simulink model "VIPL557StEnCtrl"  (R2018b)
settings: Solver=FixedStepDiscrete  StartTime=0.0  StopTime=10.0  FixedStep=0.01  RelTol=1e-3
undefined symbols (not defined in the file): data, KeSMSw4SSecRwLtStLgrstUpwdDnwdOpenPos1_Val, SecRwLtStBkReclnEn_Clear, SecRwLtStBkReclnEn_Set, SecRwLtStFwdBkwdEn_Clear, SecRwLtStFwdBkwdEn_Set, SecRwLtStLgrstInwdOtwdEn_Clear, SecRwLtStLgrstInwdOtwdEn_Set, SecRwLtStLgrstUpwdDnwdEn_Clear, SecRwLtStLgrstUpwdDnwdEn_Set, ThdRwLtStBkReclnEn_Clear, ThdRwLtStBkReclnEn_Set, ThdRwLtStFwdBkwdEn_Clear, ThdRwLtStFwdBkwdEn_Set, ZeroLEn_Clear, ZeroLEn_Set
libraries: simulink x1
settings Model: Creator=sn2xws  LastModifiedBy=sn2xws
settings Model: ModifiedHistory=|
  | 2024.7.2 V3.0.0 557模式流程V1.9
  | 2024.8.16 V3.0.1目标位置改为立即获取
  | 2024.8.22 V3.0.2 增加FirstTrig参数，智享目标位置计算改为只调用一次
  | 2024.8.30 V3.0.3 修复第一次会退出的问题
  | 2025.6.25 V3.13.0 Bug 1068643 偶发腿托及延伸先打开后动前后的问题
settings DataIOCC: SaveFormat=StructureWithTime
settings OptimizationCC: DefaultParameterBehavior=Inlined  EnhancedBackFolding=on  PassReuseOutputArgsAs=Individual arguments  ZeroExternalMemoryAtStartup=off  ZeroInternalMemoryAtStartup=off  OptimizeBlockOrder=speed  DifferentSizesBufferReuse=on  OptimizationCustomize=off
settings DebuggingCC: ParameterTunabilityLossMsg=error
settings SFSimCC: MATLABDynamicMemAlloc=off
settings RTWCC: SystemTargetFile=autosar.tlc  GenCodeOnly=on  TemplateMakefile=ert_default_tmf  Description=AUTOSAR  GenerateReport=on  IncludeHyperlinkInReport=on  LaunchReport=on  GenerateTraceInfo=on  GenerateTraceReport=on  GenerateTraceReportSl=on  GenerateTraceReportSf=on  GenerateTraceReportEml=on
settings CodeAppCC: ForceParamTrailComments=on  IgnoreCustomStorageClasses=off  OperatorAnnotations=on  SimulinkDataObjDesc=on  SFDataObjDesc=on  InsertBlockDesc=on
settings STFCustomTargetCC: TargetLangStandard=C99 (ISO)  MultiwordLength=256  ParMdlRefBuildCompliant=on  CompOptLevelCompliant=on  IncludeMdlTerminateFcn=off  CombineOutputUpdateFcns=on  SuppressErrorStatus=on  ERTCustomFileBanners=on  SupportNonFinite=off  SupportComplex=off  SupportContinuousTime=off  SupportNonInlinedSFcns=off  RemoveResetFunc=on  MATLABClassNameForMDSCustomization=Simulink.SoftwareTarget.ERTCustomization  AutosarCompliant=on  UseToolchainInfoCompliant=on  LookupTableObjectStructAxisOrder=2,1,3,4,...  LUTObjectStructOrderEvenSpacing=Size,Table,Breakpoints  SystemTargetFile=autosar.tlc
settings ERTTargetCC: TargetLangStandard=C99 (ISO)  ConcurrentExecutionCompliant=off  IncludeMdlTerminateFcn=off  SuppressErrorStatus=on  SupportNonFinite=off  SupportComplex=off  ModelStepFunctionPrototypeControlCompliant=off  CPPClassGenCompliant=off  AutosarCompliant=on  LookupTableObjectStructAxisOrder=2,1,3,4,...  LUTObjectStructOrderEvenSpacing=Size,Table,Breakpoints  InlinedParameterPlacement=NonHierarchical  ERTCustomFileTemplate=example_file_process.tlc  ERTFilePackagingFormat=Compact

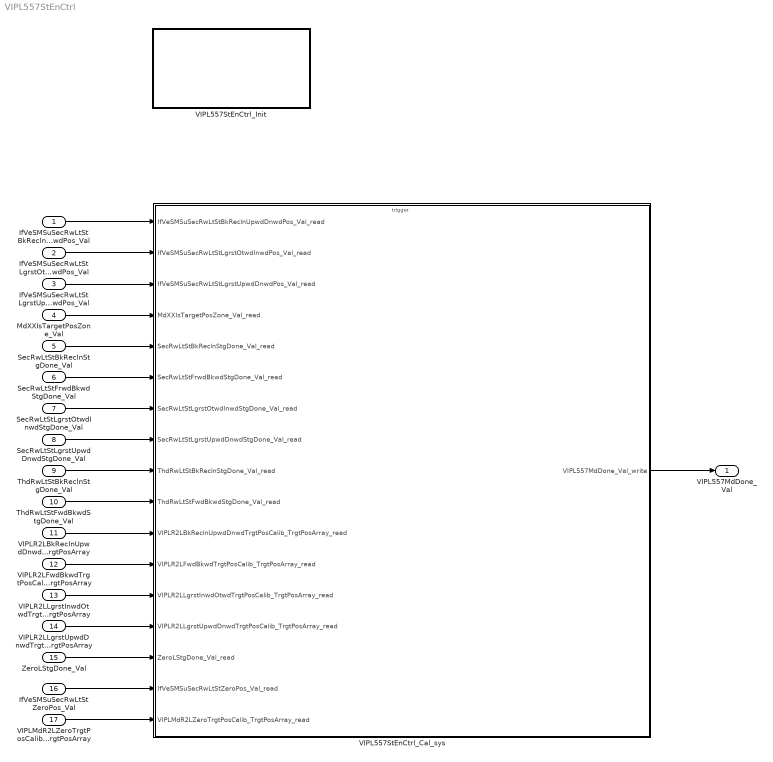
== system VIPL557StEnCtrl ==
  IfVeSMSuSecRwLtStBkReclnUpwdDnwdPos_Val : Inport  OutDataTypeStr=uint16  PortDimensions=1
  IfVeSMSuSecRwLtStLgrstOtwdInwdPos_Val : Inport  Port=2  OutDataTypeStr=uint16  PortDimensions=1
  IfVeSMSuSecRwLtStLgrstUpwdDnwdPos_Val : Inport  Port=3  OutDataTypeStr=uint16  PortDimensions=1
  MdXXIsTargetPosZone_Val : Inport  Port=4  OutDataTypeStr=uint32  PortDimensions=1
  SecRwLtStBkReclnStgDone_Val : Inport  Port=5  OutDataTypeStr=boolean  PortDimensions=1
  SecRwLtStFrwdBkwdStgDone_Val : Inport  Port=6  OutDataTypeStr=boolean  PortDimensions=1
  SecRwLtStLgrstOtwdInwdStgDone_Val : Inport  Port=7  OutDataTypeStr=boolean  PortDimensions=1
  SecRwLtStLgrstUpwdDnwdStgDone_Val : Inport  Port=8  OutDataTypeStr=boolean  PortDimensions=1
  ThdRwLtStBkReclnStgDone_Val : Inport  Port=9  OutDataTypeStr=boolean  PortDimensions=1
  ThdRwLtStFwdBkwdStgDone_Val : Inport  Port=10  OutDataTypeStr=boolean  PortDimensions=1
  VIPLR2LBkReclnUpwdDnwdTrgtPosCalib_TrgtPosArray : Inport  Description=|  Port=11  OutDataTypeStr=uint16  PortDimensions=3
      | 0:Pos
      | 1:Max
      | 2:Min
  VIPLR2LFwdBkwdTrgtPosCalib_TrgtPosArray : Inport  Description=|  Port=12  OutDataTypeStr=uint16  PortDimensions=3
      | 0:Pos
      | 1:Max
      | 2:Min
  VIPLR2LLgrstInwdOtwdTrgtPosCalib_TrgtPosArray : Inport  Description=|  Port=13  OutDataTypeStr=uint16  PortDimensions=3
      | 0:Pos
      | 1:Max
      | 2:Min
  VIPLR2LLgrstUpwdDnwdTrgtPosCalib_TrgtPosArray : Inport  Description=|  Port=14  OutDataTypeStr=uint16  PortDimensions=3
      | 0:Pos
      | 1:Max
      | 2:Min
  ZeroLStgDone_Val : Inport  Port=15  OutDataTypeStr=boolean  PortDimensions=1
  IfVeSMSuSecRwLtStZeroPos_Val : Inport  Port=16  OutDataTypeStr=uint16  PortDimensions=1
  VIPLMdR2LZeroTrgtPosCalib_TrgtPosArray : Inport  Description=|  Port=17  OutDataTypeStr=uint16  PortDimensions=3
      | 0:Pos
      | 1:Max
      | 2:Min
  VIPL557StEnCtrl_Cal_sys : Subsystem
  VIPL557StEnCtrl_Init : Subsystem
  VIPL557MdDone_Val : Outport  OutDataTypeStr=uint8  PortDimensions=1
  wires:
  IfVeSMSuSecRwLtStBkReclnUpwdDnwdPos_Val/1 -> VIPL557StEnCtrl_Cal_sys/1(IfVeSMSuSecRwLtStBkReclnUpwdDnwdPos_Val_read)
  IfVeSMSuSecRwLtStLgrstOtwdInwdPos_Val/1 -> VIPL557StEnCtrl_Cal_sys/2(IfVeSMSuSecRwLtStLgrstOtwdInwdPos_Val_read)
  IfVeSMSuSecRwLtStLgrstUpwdDnwdPos_Val/1 -> VIPL557StEnCtrl_Cal_sys/3(IfVeSMSuSecRwLtStLgrstUpwdDnwdPos_Val_read)
  MdXXIsTargetPosZone_Val/1 -> VIPL557StEnCtrl_Cal_sys/4(MdXXIsTargetPosZone_Val_read)
  SecRwLtStBkReclnStgDone_Val/1 -> VIPL557StEnCtrl_Cal_sys/5(SecRwLtStBkReclnStgDone_Val_read)
  SecRwLtStFrwdBkwdStgDone_Val/1 -> VIPL557StEnCtrl_Cal_sys/6(SecRwLtStFrwdBkwdStgDone_Val_read)
  SecRwLtStLgrstOtwdInwdStgDone_Val/1 -> VIPL557StEnCtrl_Cal_sys/7(SecRwLtStLgrstOtwdInwdStgDone_Val_read)
  SecRwLtStLgrstUpwdDnwdStgDone_Val/1 -> VIPL557StEnCtrl_Cal_sys/8(SecRwLtStLgrstUpwdDnwdStgDone_Val_read)
  ThdRwLtStBkReclnStgDone_Val/1 -> VIPL557StEnCtrl_Cal_sys/9(ThdRwLtStBkReclnStgDone_Val_read)
  ThdRwLtStFwdBkwdStgDone_Val/1 -> VIPL557StEnCtrl_Cal_sys/10(ThdRwLtStFwdBkwdStgDone_Val_read)
  VIPLR2LBkReclnUpwdDnwdTrgtPosCalib_TrgtPosArray/1 -> VIPL557StEnCtrl_Cal_sys/11(VIPLR2LBkReclnUpwdDnwdTrgtPosCalib_TrgtPosArray_read)
  VIPLR2LFwdBkwdTrgtPosCalib_TrgtPosArray/1 -> VIPL557StEnCtrl_Cal_sys/12(VIPLR2LFwdBkwdTrgtPosCalib_TrgtPosArray_read)
  VIPLR2LLgrstInwdOtwdTrgtPosCalib_TrgtPosArray/1 -> VIPL557StEnCtrl_Cal_sys/13(VIPLR2LLgrstInwdOtwdTrgtPosCalib_TrgtPosArray_read)
  VIPLR2LLgrstUpwdDnwdTrgtPosCalib_TrgtPosArray/1 -> VIPL557StEnCtrl_Cal_sys/14(VIPLR2LLgrstUpwdDnwdTrgtPosCalib_TrgtPosArray_read)
  ZeroLStgDone_Val/1 -> VIPL557StEnCtrl_Cal_sys/15(ZeroLStgDone_Val_read)
  VIPL557StEnCtrl_Cal_sys/1(VIPL557MdDone_Val_write) -> VIPL557MdDone_Val/1
  IfVeSMSuSecRwLtStZeroPos_Val/1 -> VIPL557StEnCtrl_Cal_sys/16(IfVeSMSuSecRwLtStZeroPos_Val_read)
  VIPLMdR2LZeroTrgtPosCalib_TrgtPosArray/1 -> VIPL557StEnCtrl_Cal_sys/17(VIPLMdR2LZeroTrgtPosCalib_TrgtPosArray_read)

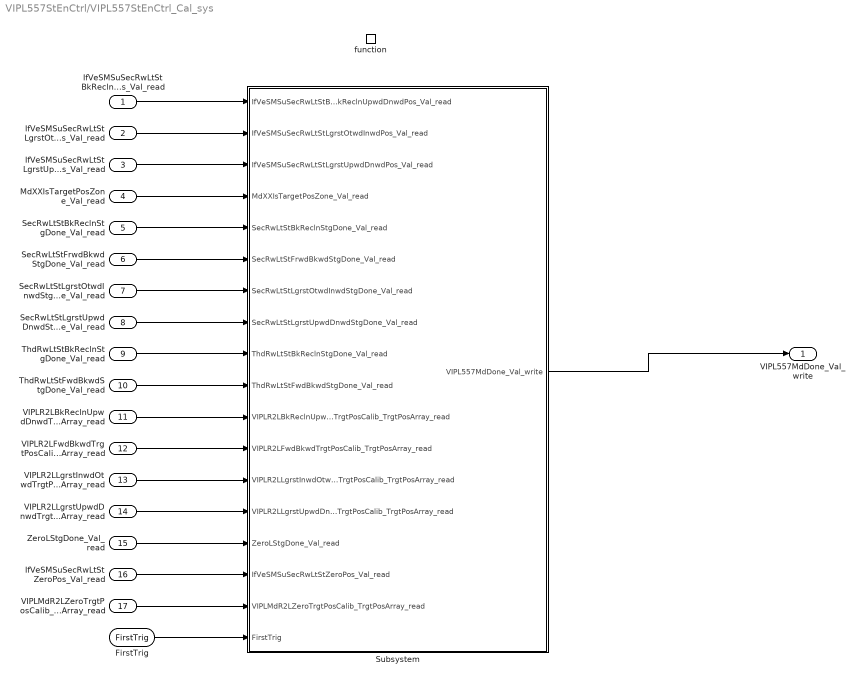
== system VIPL557StEnCtrl/VIPL557StEnCtrl_Cal_sys ==
  IfVeSMSuSecRwLtStBkReclnUpwdDnwdPos_Val_read : Inport
  IfVeSMSuSecRwLtStLgrstOtwdInwdPos_Val_read : Inport  Port=2
  IfVeSMSuSecRwLtStLgrstUpwdDnwdPos_Val_read : Inport  Port=3
  MdXXIsTargetPosZone_Val_read : Inport  Port=4
  SecRwLtStBkReclnStgDone_Val_read : Inport  Port=5
  SecRwLtStFrwdBkwdStgDone_Val_read : Inport  Port=6
  SecRwLtStLgrstOtwdInwdStgDone_Val_read : Inport  Port=7
  SecRwLtStLgrstUpwdDnwdStgDone_Val_read : Inport  Port=8
  ThdRwLtStBkReclnStgDone_Val_read : Inport  Port=9
  ThdRwLtStFwdBkwdStgDone_Val_read : Inport  Port=10
  VIPLR2LBkReclnUpwdDnwdTrgtPosCalib_TrgtPosArray_read : Inport  Port=11
  VIPLR2LFwdBkwdTrgtPosCalib_TrgtPosArray_read : Inport  Port=12
  VIPLR2LLgrstInwdOtwdTrgtPosCalib_TrgtPosArray_read : Inport  Port=13
  VIPLR2LLgrstUpwdDnwdTrgtPosCalib_TrgtPosArray_read : Inport  Port=14
  ZeroLStgDone_Val_read : Inport  Port=15
  IfVeSMSuSecRwLtStZeroPos_Val_read : Inport  Port=16
  VIPLMdR2LZeroTrgtPosCalib_TrgtPosArray_read : Inport  Port=17
  function : TriggerPort  TriggerType=function-call  IsSimulinkFunction=on  FunctionName=VIPL557StEnCtrl_Cal  VariantControl=(inherit)
  Subsystem : Subsystem
  FirstTrig : ArgIn  OutDataTypeStr=boolean  ArgumentName=FirstTrig
  VIPL557MdDone_Val_write : Outport
      settings: EnsureOutportIsVirtual=on
  wires:
  IfVeSMSuSecRwLtStBkReclnUpwdDnwdPos_Val_read/1 -> Subsystem/1(IfVeSMSuSecRwLtStBkReclnUpwdDnwdPos_Val_read)
  IfVeSMSuSecRwLtStLgrstOtwdInwdPos_Val_read/1 -> Subsystem/2(IfVeSMSuSecRwLtStLgrstOtwdInwdPos_Val_read)
  IfVeSMSuSecRwLtStLgrstUpwdDnwdPos_Val_read/1 -> Subsystem/3(IfVeSMSuSecRwLtStLgrstUpwdDnwdPos_Val_read)
  MdXXIsTargetPosZone_Val_read/1 -> Subsystem/4(MdXXIsTargetPosZone_Val_read)
  SecRwLtStBkReclnStgDone_Val_read/1 -> Subsystem/5(SecRwLtStBkReclnStgDone_Val_read)
  SecRwLtStFrwdBkwdStgDone_Val_read/1 -> Subsystem/6(SecRwLtStFrwdBkwdStgDone_Val_read)
  SecRwLtStLgrstOtwdInwdStgDone_Val_read/1 -> Subsystem/7(SecRwLtStLgrstOtwdInwdStgDone_Val_read)
  SecRwLtStLgrstUpwdDnwdStgDone_Val_read/1 -> Subsystem/8(SecRwLtStLgrstUpwdDnwdStgDone_Val_read)
  ThdRwLtStBkReclnStgDone_Val_read/1 -> Subsystem/9(ThdRwLtStBkReclnStgDone_Val_read)
  ThdRwLtStFwdBkwdStgDone_Val_read/1 -> Subsystem/10(ThdRwLtStFwdBkwdStgDone_Val_read)
  VIPLR2LBkReclnUpwdDnwdTrgtPosCalib_TrgtPosArray_read/1 -> Subsystem/11(VIPLR2LBkReclnUpwdDnwdTrgtPosCalib_TrgtPosArray_read)
  VIPLR2LFwdBkwdTrgtPosCalib_TrgtPosArray_read/1 -> Subsystem/12(VIPLR2LFwdBkwdTrgtPosCalib_TrgtPosArray_read)
  VIPLR2LLgrstInwdOtwdTrgtPosCalib_TrgtPosArray_read/1 -> Subsystem/13(VIPLR2LLgrstInwdOtwdTrgtPosCalib_TrgtPosArray_read)
  VIPLR2LLgrstUpwdDnwdTrgtPosCalib_TrgtPosArray_read/1 -> Subsystem/14(VIPLR2LLgrstUpwdDnwdTrgtPosCalib_TrgtPosArray_read)
  ZeroLStgDone_Val_read/1 -> Subsystem/15(ZeroLStgDone_Val_read)
  Subsystem/1(VIPL557MdDone_Val_write) -> VIPL557MdDone_Val_write/1
  IfVeSMSuSecRwLtStZeroPos_Val_read/1 -> Subsystem/16(IfVeSMSuSecRwLtStZeroPos_Val_read)
  VIPLMdR2LZeroTrgtPosCalib_TrgtPosArray_read/1 -> Subsystem/17(VIPLMdR2LZeroTrgtPosCalib_TrgtPosArray_read)
  FirstTrig/1 -> Subsystem/18(FirstTrig)

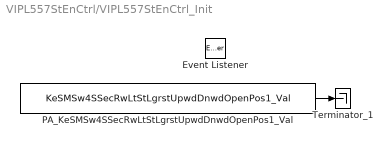
== system VIPL557StEnCtrl/VIPL557StEnCtrl_Init ==
  Event Listener : EventListener  EventName=reset
  PA_KeSMSw4SSecRwLtStLgrstUpwdDnwdOpenPos1_Val : Constant  Value=KeSMSw4SSecRwLtStLgrstUpwdDnwdOpenPos1_Val
  Terminator_1 : Terminator
  wires:
  PA_KeSMSw4SSecRwLtStLgrstUpwdDnwdOpenPos1_Val/1 -> Terminator_1/1

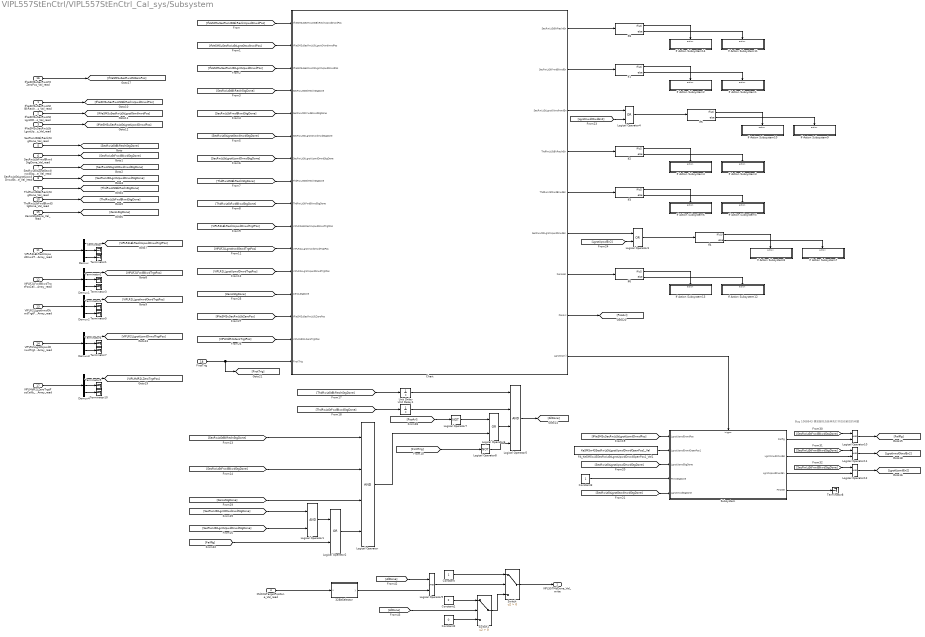
== system VIPL557StEnCtrl/VIPL557StEnCtrl_Cal_sys/Subsystem ==
  note: Bug 1068643 偶发腿托及延伸先打开后动前后的问题
  IfVeSMSuSecRwLtStBkReclnUpwdDnwdPos_Val_read : Inport
  IfVeSMSuSecRwLtStLgrstOtwdInwdPos_Val_read : Inport  Port=2
  IfVeSMSuSecRwLtStLgrstUpwdDnwdPos_Val_read : Inport  Port=3
  MdXXIsTargetPosZone_Val_read : Inport  Port=4
  SecRwLtStBkReclnStgDone_Val_read : Inport  Port=5
  SecRwLtStFrwdBkwdStgDone_Val_read : Inport  Port=6
  SecRwLtStLgrstOtwdInwdStgDone_Val_read : Inport  Port=7
  SecRwLtStLgrstUpwdDnwdStgDone_Val_read : Inport  Port=8
  ThdRwLtStBkReclnStgDone_Val_read : Inport  Port=9
  ThdRwLtStFwdBkwdStgDone_Val_read : Inport  Port=10
  VIPLR2LBkReclnUpwdDnwdTrgtPosCalib_TrgtPosArray_read : Inport  Port=11
  VIPLR2LFwdBkwdTrgtPosCalib_TrgtPosArray_read : Inport  Port=12
  VIPLR2LLgrstInwdOtwdTrgtPosCalib_TrgtPosArray_read : Inport  Port=13
  VIPLR2LLgrstUpwdDnwdTrgtPosCalib_TrgtPosArray_read : Inport  Port=14
  ZeroLStgDone_Val_read : Inport  Port=15
  IfVeSMSuSecRwLtStZeroPos_Val_read : Inport  Port=16
  VIPLMdR2LZeroTrgtPosCalib_TrgtPosArray_read : Inport  Port=17
  FirstTrig : Inport  Port=18
  32BitSelector : Subsystem  mask(32 Bit Selector){BitNum=9}
      mask prompts: BitNum "Select Bit Number"
      mask help: Allows selection of a particular bit (0-31) out of a packed word up to 32 bits long. Output will be true if the bit number selected via the mask parameter is equal to one.
      mask TypeOptions BitNum: 0 | 1 | 2 | 3 | 4 | 5 | 6 | 7 | 8 | 9 | 10 | 11 | 12 | 13 | 14 | 15 | 16 | 17 | 18 | 19 | 20 | 21 | 22 | 23 | 24 | 25 | 26 | 27 | 28 | 29 | 30 | 31
      mask Display:
      | text(0.5, 0.8,'BIT','horizontalAlignment','center')
      | text(0.5, 0.5,'SELECTOR','horizontalAlignment','center')
      | text(0.5, 0.2,['-- Bit ',char(get_param(gcb,'BitNum')),' --'],'horizontalAlignment','center')
  Chart : Stateflow chart  TreatAsAtomicUnit=on
  Constant : Constant  OutDataTypeStr=uint8
  Constant1 : Constant  Value=2  OutDataTypeStr=uint8
  Constant2 : Constant  Value=0  OutDataTypeStr=uint8
  Constant3 : Constant  OutDataTypeStr=boolean
  Demux{,1..4} (5 alike) : Demux  Outputs=3
  If Action Subsystem1 : Subsystem  TreatAsAtomicUnit=on
  If Action Subsystem10 : Subsystem  TreatAsAtomicUnit=on
  If Action Subsystem11 : Subsystem  TreatAsAtomicUnit=on
  If Action Subsystem12 : Subsystem  TreatAsAtomicUnit=on
  If Action Subsystem13 : Subsystem  TreatAsAtomicUnit=on
  If Action Subsystem14 : Subsystem  TreatAsAtomicUnit=on
  If Action Subsystem2 : Subsystem  TreatAsAtomicUnit=on
  If Action Subsystem3 : Subsystem  TreatAsAtomicUnit=on
  If Action Subsystem4 : Subsystem  TreatAsAtomicUnit=on
  If Action Subsystem5 : Subsystem  TreatAsAtomicUnit=on
  If Action Subsystem6 : Subsystem  TreatAsAtomicUnit=on
  If Action Subsystem7 : Subsystem  TreatAsAtomicUnit=on
  If Action Subsystem8 : Subsystem  TreatAsAtomicUnit=on
  If Action Subsystem9 : Subsystem  TreatAsAtomicUnit=on
  If{1..6,8} (7 alike) : If  IfExpression=u1
  Logical Operator : Logic  Inputs=4  AllPortsSameDT=off  OutDataTypeStr=boolean
  Logical Operator{1,9..12} (5 alike) : Logic  AllPortsSameDT=off  OutDataTypeStr=boolean
  Logical Operator{2..4,6} (4 alike) : Logic  Operator=OR  AllPortsSameDT=off  OutDataTypeStr=boolean
  Logical Operator5 : Logic  Inputs=4  AllPortsSameDT=off  OutDataTypeStr=boolean
  Logical Operator7 : Logic  Operator=NOT  AllPortsSameDT=off  OutDataTypeStr=boolean
  Logical Operator8 : Logic  Operator=NOT  AllPortsSameDT=off  OutDataTypeStr=boolean
  PA_KeSMSw4SSecRwLtStLgrstUpwdDnwdOpenPos1_Val1 : Constant  Value=KeSMSw4SSecRwLtStLgrstUpwdDnwdOpenPos1_Val
  Subsystem : Subsystem
  Switch : Switch  Criteria=u2 > Threshold
  Switch1 : Switch  Criteria=u2 > Threshold
  Terminator{,1..10} (11 alike) : Terminator
  Unit Delay : UnitDelay  SampleTime=-1
  Unit Delay1 : UnitDelay  SampleTime=-1
  VIPL557MdDone_Val_write : Outport
      settings: EnsureOutportIsVirtual=on
  wires:
  Switch/1 -> VIPL557MdDone_Val_write/1
  IfVeSMSuSecRwLtStBkReclnUpwdDnwdPos_Val_read/1 -> [IfVeSMSuSecRwLtStBkReclnUpwdDnwdPos]
  IfVeSMSuSecRwLtStLgrstOtwdInwdPos_Val_read/1 -> [IfVeSMSuSecRwLtStLgrstOtwdInwdPos]
  ThdRwLtStFwdBkwdStgDone_Val_read/1 -> [ThdRwLtStFwdBkwdStgDone]
  IfVeSMSuSecRwLtStLgrstUpwdDnwdPos_Val_read/1 -> [IfVeSMSuSecRwLtStLgrstUpwdDnwdPos]
  ThdRwLtStBkReclnStgDone_Val_read/1 -> [ThdRwLtStBkReclnStgDone]
  SecRwLtStFrwdBkwdStgDone_Val_read/1 -> [SecRwLtStFrwdBkwdStgDone]
  SecRwLtStLgrstOtwdInwdStgDone_Val_read/1 -> [SecRwLtStLgrstOtwdInwdStgDone]
  SecRwLtStLgrstUpwdDnwdStgDone_Val_read/1 -> [SecRwLtStLgrstUpwdDnwdStgDone]
  SecRwLtStBkReclnStgDone_Val_read/1 -> [SecRwLtStBkReclnStgDone]
  ZeroLStgDone_Val_read/1 -> [ZeroLStgDone]
  Demux/3 -> Terminator1/1
  VIPLR2LBkReclnUpwdDnwdTrgtPosCalib_TrgtPosArray_read/1 -> Demux/1
  Demux3/2 -> Terminator6/1
  Demux1/3 -> Terminator3/1
  Demux1/1 -> [VIPLR2LFwdBkwdTrgtPos]
  Demux1/2 -> Terminator2/1
  Demux2/3 -> Terminator5/1
  Demux/2 -> Terminator/1
  Demux2/2 -> Terminator4/1
  Demux/1 -> [VIPLR2LBkReclnUpwdDnwdTrgtPos]
  Demux3/3 -> Terminator7/1
  Demux2/1 -> [VIPLR2LLgrstInwdOtwdTrgtPos]
  Demux3/1 -> [VIPLR2LLgrstUpwdDnwdTrgtPos]
  VIPLR2LFwdBkwdTrgtPosCalib_TrgtPosArray_read/1 -> Demux1/1
  VIPLR2LLgrstUpwdDnwdTrgtPosCalib_TrgtPosArray_read/1 -> Demux3/1
  VIPLR2LLgrstInwdOtwdTrgtPosCalib_TrgtPosArray_read/1 -> Demux2/1
  [SecRwLtStLgrstUpwdDnwdStgDone] -> Logical Operator1/2
  [SecRwLtStFrwdBkwdStgDone] -> Logical Operator/2
  If5/2 -> If Action Subsystem9/Action
  [LgrstInwdOtwdEn2] -> Logical Operator4/2
  If1/1 -> If Action Subsystem2/Action
  [IfVeSMSuSecRwLtStLgrstUpwdDnwdPos] -> Chart/3(IfVeSMSuSecRwLtStLgrstUpwdDnwdPos)
  If5/1 -> If Action Subsystem10/Action
  Logical Operator3/1 -> If4/1
  Subsystem/4(FtrstEn) -> Terminator8/1
  If4/2 -> If Action Subsystem7/Action
  If3/2 -> If Action Subsystem5/Action
  [LgrstUpwdEn2] -> Logical Operator3/2
  [SecRwLtStLgrstUpwdDnwdStgDone] -> Subsystem/3(LgrstUpwdStgDone)
  Chart/3(SecRwLtStLgrstOtwdInwdEn) -> Logical Operator4/1
  Chart/1(SecRwLtStBkReclnEn) -> If8/1
  Chart/6(SecRwLtStLgrstUpwdDnwdEn) -> Logical Operator3/1
  If2/1 -> If Action Subsystem4/Action
  If3/1 -> If Action Subsystem6/Action
  Logical Operator1/1 -> Logical Operator2/1
  [ThdRwLtStFwdBkwdStgDone] -> Chart/9(ThdRwLtStFwdBkwdStgDone)
  Logical Operator4/1 -> If5/1
  Chart/5(ThdRwLtStFwdBkwdEn) -> If3/1
  If1/2 -> If Action Subsystem1/Action
  Chart/2(SecRwLtStFrwdBkwdEn) -> If1/1
  PA_KeSMSw4SSecRwLtStLgrstUpwdDnwdOpenPos1_Val1/1 -> Subsystem/2(LgrstUpwdDnwdOpenPos1)
  Chart/9(LgrstOpn()) -> Subsystem/Trigger
  Chart/4(ThdRwLtStBkReclnEn) -> If2/1
  If8/1 -> If Action Subsystem14/Action
  If2/2 -> If Action Subsystem3/Action
  [Failflg] -> Logical Operator2/2
  [VIPLR2LLgrstInwdOtwdTrgtPos] -> Chart/11(VIPLR2LLgrstInwdOtwdTrgtPos)
  [VIPLR2LLgrstUpwdDnwdTrgtPos] -> Chart/12(VIPLR2LLgrstUpwdDnwdTrgtPos)
  [IfVeSMSuSecRwLtStLgrstOtwdInwdPos] -> Chart/2(IfVeSMSuSecRwLtStLgrstOtwdInwdPos)
  [SecRwLtStFrwdBkwdStgDone] -> Chart/5(SecRwLtStFrwdBkwdStgDone)
  [SecRwLtStBkReclnStgDone] -> Chart/4(SecRwLtStBkReclnStgDone)
  [SecRwLtStLgrstOtwdInwdStgDone] -> Logical Operator1/1
  [IfVeSMSuSecRwLtStLgrstUpwdDnwdPos] -> Subsystem/1(LgrstUpwdDnwdPos)
  If4/1 -> If Action Subsystem8/Action
  [VIPLR2LBkReclnUpwdDnwdTrgtPos] -> Chart/10(VIPLR2LBkReclnUpwdDnwdTrgtPos)
  Constant3/1 -> Subsystem/4(FtrstStgDone)
  [SecRwLtStLgrstUpwdDnwdStgDone] -> Chart/7(SecRwLtStLgrstUpwdDnwdStgDone)
  [ThdRwLtStBkReclnStgDone] -> Chart/8(ThdRwLtStBkReclnStgDone)
  [SecRwLtStBkReclnStgDone] -> Logical Operator/1
  [SecRwLtStLgrstOtwdInwdStgDone] -> Chart/6(SecRwLtStLgrstOtwdInwdStgDone)
  [SecRwLtStLgrstOtwdInwdStgDone] -> Subsystem/5(LgrstInwdStgDone)
  If8/2 -> If Action Subsystem11/Action
  [IfVeSMSuSecRwLtStBkReclnUpwdDnwdPos] -> Chart/1(IfVeSMSuSecRwLtStBkReclnUpwdDnwdPos)
  MdXXIsTargetPosZone_Val_read/1 -> 32BitSelector/1(x)
  Constant2/1 -> Switch1/3
  [AllDone] -> Switch1/2
  [AllDone] -> Logical Operator9/1
  Constant/1 -> Switch/1
  Logical Operator9/1 -> Switch/2
  Constant1/1 -> Switch1/1
  Switch1/1 -> Switch/3
  32BitSelector/1(y) -> Logical Operator9/2
  [ZeroLStgDone] -> Chart/13(ZeroLStgDone)
  IfVeSMSuSecRwLtStZeroPos_Val_read/1 -> [IfVeSMSuSecRwLtStZeroPos]
  VIPLMdR2LZeroTrgtPosCalib_TrgtPosArray_read/1 -> Demux4/1
  Demux4/1 -> [VIPLMdR2LZeroTrgtPos]
  Demux4/3 -> Terminator10/1
  Demux4/2 -> Terminator9/1
  [IfVeSMSuSecRwLtStZeroPos] -> Chart/14(IfVeSMSuSecRwLtStZeroPos)
  [VIPLMdR2LZeroTrgtPos] -> Chart/15(VIPLMdR2LZeroTrgtPos)
  Chart/7(ZeroLEn) -> If6/1
  If6/1 -> If Action Subsystem13/Action
  If6/2 -> If Action Subsystem12/Action
  Chart/8(PosAvl) -> [PosAvl]
  Logical Operator2/1 -> Logical Operator/4
  [ZeroLStgDone] -> Logical Operator/3
  [ThdRwLtStBkReclnStgDone] -> Unit Delay/1
  [ThdRwLtStFwdBkwdStgDone] -> Unit Delay1/1
  Logical Operator5/1 -> [AllDone]
  [PosAvl] -> Logical Operator7/1
  Logical Operator6/1 -> Logical Operator5/3
  Logical Operator/1 -> Logical Operator6/2
  Unit Delay/1 -> Logical Operator5/1
  Unit Delay1/1 -> Logical Operator5/2
  Logical Operator7/1 -> Logical Operator6/1
  FirstTrig/1 -> [FirstTrig], Chart/16(FirstTrig)
  Logical Operator8/1 -> Logical Operator5/4
  [FirstTrig] -> Logical Operator8/1
  Logical Operator10/1 -> [Failflg]
  Subsystem/1(Failflg) -> Logical Operator10/2
  [SecRwLtStFrwdBkwdStgDone] -> Logical Operator10/1
  [SecRwLtStFrwdBkwdStgDone] -> Logical Operator11/1
  Logical Operator11/1 -> [LgrstInwdOtwdEn2]
  Subsystem/2(LgrstInwdOtwdEn) -> Logical Operator11/2
  Logical Operator12/1 -> [LgrstUpwdEn2]
  [SecRwLtStFrwdBkwdStgDone] -> Logical Operator12/1
  Subsystem/3(LgrstUpwdDnwdEn) -> Logical Operator12/2

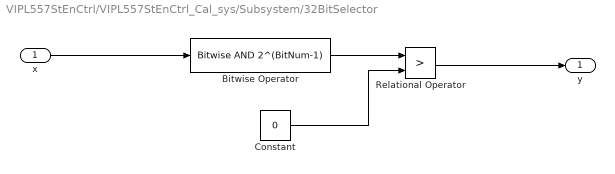
== system VIPL557StEnCtrl/VIPL557StEnCtrl_Cal_sys/Subsystem/32BitSelector ==
  x : Inport
  Bitwise Operator : simulink/Logic and Bit Operations/Bitwise Operator  logicop=AND  UseBitMask=on  BitMask=2^(BitNum-1)  BitMaskRealWorld=Stored Integer
  Constant : Constant  Value=0  OutDataTypeStr=uint32
  Relational Operator : RelationalOperator  Operator=>  OutDataTypeStr=boolean  RndMeth=Simplest
  y : Outport
  wires:
  Relational Operator/1 -> y/1
  Constant/1 -> Relational Operator/2
  x/1 -> Bitwise Operator/1
  Bitwise Operator/1 -> Relational Operator/1

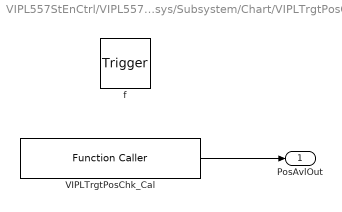
== system VIPL557StEnCtrl/VIPL557StEnCtrl_Cal_sys/Subsystem/Chart/VIPLTrgtPosChk ==
  f : TriggerPort  TriggerType=function-call  VariantControl=(inherit)
      settings: CopyFcn=Stateflow.SLINSF.SimulinkMan.removeBlockPreDeleteFcn  PreDeleteFcn=Stateflow.SLINSF.SimulinkMan.unsafePredeleteFcn
  VIPLTrgtPosChk_Cal : FunctionCaller  FunctionPrototype=PosAvl = VIPLTrgtPosChk_Cal()  OutputArgumentSpecifications=uint8(1)
  PosAvlOut : Outport
  wires:
  VIPLTrgtPosChk_Cal/1 -> PosAvlOut/1

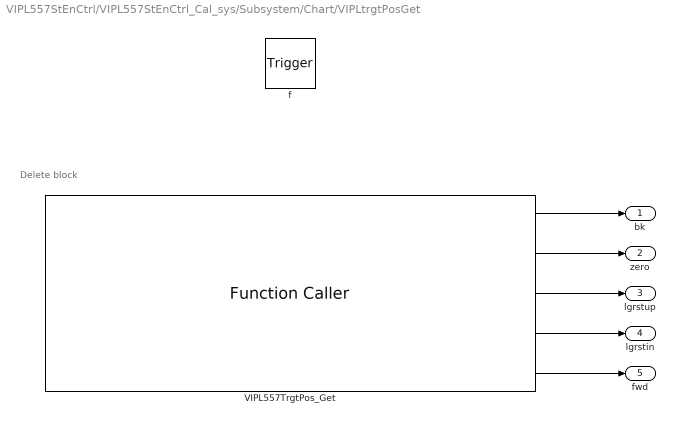
== system VIPL557StEnCtrl/VIPL557StEnCtrl_Cal_sys/Subsystem/Chart/VIPLtrgtPosGet ==
  note: Delete block
  f : TriggerPort  TriggerType=function-call  VariantControl=(inherit)
      settings: CopyFcn=Stateflow.SLINSF.SimulinkMan.removeBlockPreDeleteFcn  PreDeleteFcn=Stateflow.SLINSF.SimulinkMan.unsafePredeleteFcn
  VIPL557TrgtPos_Get : FunctionCaller  FunctionPrototype=[SecRwLtStBkReclnTrgtPos,SecRwLtStZeroTrgtPos,SecRwLtStLgrstUpwdDnwdTrgtPos,SecRwLtStLgrstInwdOtwdTrgtPos,SecRwLtStFwdBkwdTrgtPos] = VIPL557TrgtPos_Get()  OutputArgumentSpecifications=uint16(1), uint16(1), uint16(1), uint16(1), uint16(1)
  bk : Outport
  zero : Outport  Port=2
  lgrstup : Outport  Port=3
  lgrstin : Outport  Port=4
  fwd : Outport  Port=5
  wires:
  VIPL557TrgtPos_Get/1 -> bk/1
  VIPL557TrgtPos_Get/3 -> lgrstup/1
  VIPL557TrgtPos_Get/2 -> zero/1
  VIPL557TrgtPos_Get/4 -> lgrstin/1
  VIPL557TrgtPos_Get/5 -> fwd/1

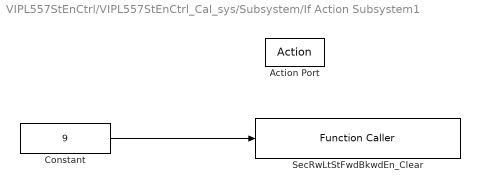
== system VIPL557StEnCtrl/VIPL557StEnCtrl_Cal_sys/Subsystem/If Action Subsystem1 ==
  Action Port : ActionPort  ActionType=else
  Constant : Constant  Value=9  OutDataTypeStr=uint8
  SecRwLtStFwdBkwdEn_Clear : FunctionCaller  FunctionPrototype=SecRwLtStFwdBkwdEn_Clear(data)  InputArgumentSpecifications=uint8(1)
  wires:
  Constant/1 -> SecRwLtStFwdBkwdEn_Clear/1

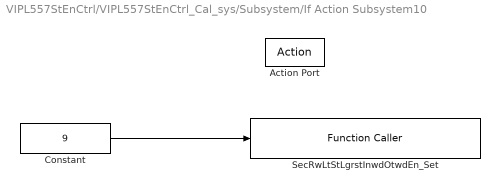
== system VIPL557StEnCtrl/VIPL557StEnCtrl_Cal_sys/Subsystem/If Action Subsystem10 ==
  Action Port : ActionPort  ActionType=then
  Constant : Constant  Value=9  OutDataTypeStr=uint8
  SecRwLtStLgrstInwdOtwdEn_Set : FunctionCaller  FunctionPrototype=SecRwLtStLgrstInwdOtwdEn_Set(data)  InputArgumentSpecifications=uint8(1)
  wires:
  Constant/1 -> SecRwLtStLgrstInwdOtwdEn_Set/1

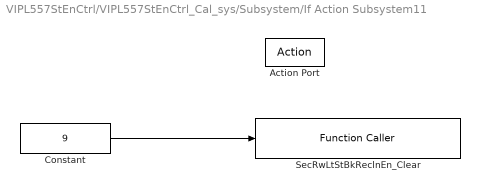
== system VIPL557StEnCtrl/VIPL557StEnCtrl_Cal_sys/Subsystem/If Action Subsystem11 ==
  Action Port : ActionPort  ActionType=else
  Constant : Constant  Value=9  OutDataTypeStr=uint8
  SecRwLtStBkReclnEn_Clear : FunctionCaller  FunctionPrototype=SecRwLtStBkReclnEn_Clear(data)  InputArgumentSpecifications=uint8(1)
  wires:
  Constant/1 -> SecRwLtStBkReclnEn_Clear/1

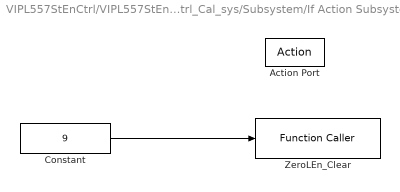
== system VIPL557StEnCtrl/VIPL557StEnCtrl_Cal_sys/Subsystem/If Action Subsystem12 ==
  Action Port : ActionPort  ActionType=else
  Constant : Constant  Value=9  OutDataTypeStr=uint8
  ZeroLEn_Clear : FunctionCaller  FunctionPrototype=ZeroLEn_Clear(data)  InputArgumentSpecifications=uint8(1)
  wires:
  Constant/1 -> ZeroLEn_Clear/1

== system VIPL557StEnCtrl/VIPL557StEnCtrl_Cal_sys/Subsystem/If Action Subsystem13 ==
  Action Port : ActionPort  ActionType=then
  Constant : Constant  Value=9  OutDataTypeStr=uint8
  ZeroLEn_Set : FunctionCaller  FunctionPrototype=ZeroLEn_Set(data)  InputArgumentSpecifications=uint8(1)
  wires:
  Constant/1 -> ZeroLEn_Set/1

== system VIPL557StEnCtrl/VIPL557StEnCtrl_Cal_sys/Subsystem/If Action Subsystem14 ==
  Action Port : ActionPort  ActionType=then
  Constant : Constant  Value=9  OutDataTypeStr=uint8
  SecRwLtStBkReclnEn_Set : FunctionCaller  FunctionPrototype=SecRwLtStBkReclnEn_Set(data)  InputArgumentSpecifications=uint8(1)
  wires:
  Constant/1 -> SecRwLtStBkReclnEn_Set/1

== system VIPL557StEnCtrl/VIPL557StEnCtrl_Cal_sys/Subsystem/If Action Subsystem2 ==
  Action Port : ActionPort  ActionType=then
  Constant : Constant  Value=9  OutDataTypeStr=uint8
  SecRwLtStFwdBkwdEn_Set : FunctionCaller  FunctionPrototype=SecRwLtStFwdBkwdEn_Set(data)  InputArgumentSpecifications=uint8(1)
  wires:
  Constant/1 -> SecRwLtStFwdBkwdEn_Set/1

== system VIPL557StEnCtrl/VIPL557StEnCtrl_Cal_sys/Subsystem/If Action Subsystem3 ==
  Action Port : ActionPort  ActionType=else
  Constant : Constant  Value=9  OutDataTypeStr=uint8
  ThdRwLtStBkReclnEn_Clear : FunctionCaller  FunctionPrototype=ThdRwLtStBkReclnEn_Clear(data)  InputArgumentSpecifications=uint8(1)
  wires:
  Constant/1 -> ThdRwLtStBkReclnEn_Clear/1

== system VIPL557StEnCtrl/VIPL557StEnCtrl_Cal_sys/Subsystem/If Action Subsystem4 ==
  Action Port : ActionPort  ActionType=then
  Constant : Constant  Value=9  OutDataTypeStr=uint8
  ThdRwLtStBkReclnEn_Set : FunctionCaller  FunctionPrototype=ThdRwLtStBkReclnEn_Set(data)  InputArgumentSpecifications=uint8(1)
  wires:
  Constant/1 -> ThdRwLtStBkReclnEn_Set/1

== system VIPL557StEnCtrl/VIPL557StEnCtrl_Cal_sys/Subsystem/If Action Subsystem5 ==
  Action Port : ActionPort  ActionType=else
  Constant : Constant  Value=9  OutDataTypeStr=uint8
  ThdRwLtStFwdBkwdEn_Clear : FunctionCaller  FunctionPrototype=ThdRwLtStFwdBkwdEn_Clear(data)  InputArgumentSpecifications=uint8(1)
  wires:
  Constant/1 -> ThdRwLtStFwdBkwdEn_Clear/1

== system VIPL557StEnCtrl/VIPL557StEnCtrl_Cal_sys/Subsystem/If Action Subsystem6 ==
  Action Port : ActionPort  ActionType=then
  Constant : Constant  Value=9  OutDataTypeStr=uint8
  ThdRwLtStFwdBkwdEn_Set : FunctionCaller  FunctionPrototype=ThdRwLtStFwdBkwdEn_Set(data)  InputArgumentSpecifications=uint8(1)
  wires:
  Constant/1 -> ThdRwLtStFwdBkwdEn_Set/1

== system VIPL557StEnCtrl/VIPL557StEnCtrl_Cal_sys/Subsystem/If Action Subsystem7 ==
  Action Port : ActionPort  ActionType=else
  Constant : Constant  Value=9  OutDataTypeStr=uint8
  SecRwLtStLgrstUpwdDnwdEn_Clear : FunctionCaller  FunctionPrototype=SecRwLtStLgrstUpwdDnwdEn_Clear(data)  InputArgumentSpecifications=uint8(1)
  wires:
  Constant/1 -> SecRwLtStLgrstUpwdDnwdEn_Clear/1

== system VIPL557StEnCtrl/VIPL557StEnCtrl_Cal_sys/Subsystem/If Action Subsystem8 ==
  Action Port : ActionPort  ActionType=then
  Constant : Constant  Value=9  OutDataTypeStr=uint8
  SecRwLtStLgrstUpwdDnwdEn_Set : FunctionCaller  FunctionPrototype=SecRwLtStLgrstUpwdDnwdEn_Set(data)  InputArgumentSpecifications=uint8(1)
  wires:
  Constant/1 -> SecRwLtStLgrstUpwdDnwdEn_Set/1

== system VIPL557StEnCtrl/VIPL557StEnCtrl_Cal_sys/Subsystem/If Action Subsystem9 ==
  Action Port : ActionPort  ActionType=else
  Constant : Constant  Value=9  OutDataTypeStr=uint8
  SecRwLtStLgrstInwdOtwdEn_Clear : FunctionCaller  FunctionPrototype=SecRwLtStLgrstInwdOtwdEn_Clear(data)  InputArgumentSpecifications=uint8(1)
  wires:
  Constant/1 -> SecRwLtStLgrstInwdOtwdEn_Clear/1

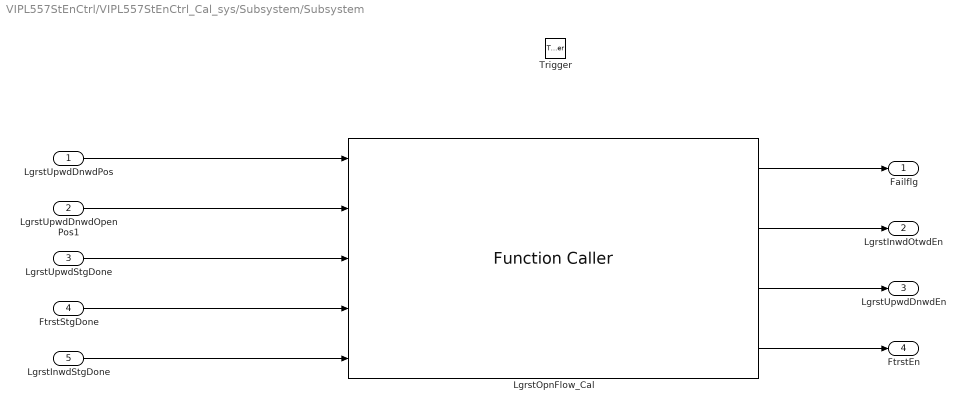
== system VIPL557StEnCtrl/VIPL557StEnCtrl_Cal_sys/Subsystem/Subsystem ==
  LgrstUpwdDnwdPos : Inport
  LgrstUpwdDnwdOpenPos1 : Inport  Port=2
  LgrstUpwdStgDone : Inport  Port=3
  FtrstStgDone : Inport  Port=4
  LgrstInwdStgDone : Inport  Port=5
  Trigger : TriggerPort  TriggerType=function-call  VariantControl=Variant  PortDimensions=1
  LgrstOpnFlow_Cal : FunctionCaller  FunctionPrototype=[Failflg,LgrstInwdOtwdEn,LgrstUpwdDnwdEn,FtrstEn] = LgrstOpnFlow_Cal(LgrstUpwdDnwdPos,LgrstUpwdDnwdOpenPos1,LgrstUpwdStgDone,FtrstStgDone,LgrstInwdStgDone)  InputArgumentSpecifications=uint16(1), uint16(1), boolean(true), boolean(true), boolean(true)  OutputArgumentSpecifications=boolean(true), boolean(true), boolean(true), boolean(true)
  Failflg : Outport
  LgrstInwdOtwdEn : Outport  Port=2
  LgrstUpwdDnwdEn : Outport  Port=3
  FtrstEn : Outport  Port=4
  wires:
  LgrstOpnFlow_Cal/2 -> LgrstInwdOtwdEn/1
  LgrstUpwdDnwdPos/1 -> LgrstOpnFlow_Cal/1
  LgrstOpnFlow_Cal/3 -> LgrstUpwdDnwdEn/1
  FtrstStgDone/1 -> LgrstOpnFlow_Cal/4
  LgrstUpwdStgDone/1 -> LgrstOpnFlow_Cal/3
  LgrstOpnFlow_Cal/4 -> FtrstEn/1
  LgrstInwdStgDone/1 -> LgrstOpnFlow_Cal/5
  LgrstUpwdDnwdOpenPos1/1 -> LgrstOpnFlow_Cal/2
  LgrstOpnFlow_Cal/1 -> Failflg/1

== stateflow chart VIPL557StEnCtrl/VIPL557StEnCtrl_Cal_sys/Subsystem/Chart ==
  state PosAvlOut=VIPLTrgtPosChk [function]
  state [bk,zero,lgrstup,lgrstin,fwd]=VIPLtrgtPosGet [function]
  (default) -> (junction 157) : {
      | ThdRwLtStBkReclnEn = 0;
      | SecRwLtStBkReclnEn = 0;
      | SecRwLtStFrwdBkwdEn = 0;
      | SecRwLtStLgrstOtwdInwdEn = 0;
      | SecRwLtStLgrstUpwdDnwdEn = 0;
      | ThdRwLtStFwdBkwdEn = 0;
      | ZeroLEn = 0;
      | }
  (junction 157) -> (junction 159) [order 1] : [FirstTrig]
  (junction 157) -> (junction 163) [order 2]
  (junction 159) -> (junction 161) : {PosAvl = 0;}
  (junction 161) -> (junction 163)
  (junction 163) -> (junction 1)
  (junction 1) -> (junction 22) [order 1] : [ThdRwLtStBkReclnStgDone]
  (junction 1) -> (junction 26) [order 2] : {ThdRwLtStBkReclnEn = 1;}
  (junction 22) -> (junction 24)
  (junction 24) -> (junction 26)
  (junction 26) -> (junction 29)
  (junction 29) -> (junction 31) [order 1] : [ThdRwLtStFwdBkwdStgDone]
  (junction 29) -> (junction 35) [order 2] : {
      | ThdRwLtStFwdBkwdEn = 1;
      | }
  (junction 31) -> (junction 33)
  (junction 33) -> (junction 35)
  (junction 35) -> (junction 92)
  (junction 92) -> (junction 100) [order 1] : [ThdRwLtStBkReclnStgDone&&ThdRwLtStFwdBkwdStgDone]
  (junction 100) -> (junction 166) [order 1] : [!PosAvl]
  (junction 92) -> (junction 95) [order 2]
  (junction 100) -> (junction 170) [order 2]
  (junction 166) -> (junction 168) : {PosAvl = VIPLTrgtPosChk();}
  (junction 168) -> (junction 170)
  (junction 170) -> (junction 129)
  (junction 129) -> (junction 105) [order 1] : [PosAvl]
  (junction 129) -> (junction 109) [order 2]
  (junction 105) -> (junction 38) : {[bktrgt,zerotrgt,lgrstuptrgt,lgrstintrgt,fwdtrgt]=VIPLtrgtPosGet();}
  (junction 38) -> (junction 40) [order 1] : [IfVeSMSuSecRwLtStBkReclnUpwdDnwdPos>bktrgt&&!SecRwLtStBkReclnStgDone]
  (junction 38) -> (junction 44) [order 2]
  (junction 40) -> (junction 42) : {SecRwLtStBkReclnEn = 1;}
  (junction 42) -> (junction 44)
  (junction 44) -> (junction 47)
  (junction 47) -> (junction 49) [order 1] : [IfVeSMSuSecRwLtStLgrstOtwdInwdPos >lgrstintrgt &&!SecRwLtStLgrstOtwdInwdStgDone]
  (junction 47) -> (junction 53) [order 2]
  (junction 49) -> (junction 51) : {SecRwLtStLgrstOtwdInwdEn = 1;}
  (junction 51) -> (junction 53)
  (junction 53) -> (junction 56)
  (junction 56) -> (junction 58) [order 1] : [IfVeSMSuSecRwLtStLgrstUpwdDnwdPos >lgrstuptrgt && !SecRwLtStLgrstUpwdDnwdStgDone]
  (junction 56) -> (junction 62) [order 2]
  (junction 58) -> (junction 60) : {SecRwLtStLgrstUpwdDnwdEn = 1;}
  (junction 60) -> (junction 62)
  (junction 62) -> (junction 111)
  (junction 111) -> (junction 113) [order 1] : [IfVeSMSuSecRwLtStZeroPos >zerotrgt && !ZeroLStgDone]
  (junction 111) -> (junction 117) [order 2]
  (junction 113) -> (junction 115) : {ZeroLEn = 1;}
  (junction 115) -> (junction 117)
  (junction 117) -> (junction 65)
  (junction 65) -> (junction 67) [order 1] : [(IfVeSMSuSecRwLtStBkReclnUpwdDnwdPos<=bktrgt||SecRwLtStBkReclnStgDone)&&...
      | (IfVeSMSuSecRwLtStLgrstOtwdInwdPos <=lgrstintrgt ||SecRwLtStLgrstOtwdInwdStgDone) &&...
      | (IfVeSMSuSecRwLtStLgrstUpwdDnwdPos <=lgrstuptrgt ||SecRwLtStLgrstUpwdDnwdStgDone)&&...
      | (IfVeSMSuSecRwLtStZeroPos <= zerotrgt || ZeroLStgDone)]
  (junction 67) -> (junction 69) [order 1] : [SecRwLtStFrwdBkwdStgDone]
  (junction 69) -> (junction 76) [order 1] : [SecRwLtStBkReclnStgDone]
  (junction 65) -> (junction 87) [order 2]
  (junction 67) -> (junction 73) [order 2] : {SecRwLtStFrwdBkwdEn =1;}
  (junction 69) -> (junction 71) [order 2] : {SecRwLtStBkReclnEn = 1;}
  (junction 76) -> (junction 78)
  (junction 78) -> (junction 71)
  (junction 71) -> (junction 132)
  (junction 132) -> (junction 134) [order 1] : [ZeroLStgDone]
  (junction 132) -> (junction 138) [order 2] : {ZeroLEn = 1;}
  (junction 134) -> (junction 136)
  (junction 136) -> (junction 138)
  (junction 138) -> (junction 81) : {LgrstOpn;}
  (junction 109) -> (junction 95)
  (junction 87) -> (junction 109)
  (junction 73) -> (junction 87)
  (junction 81) -> (junction 73)
  (junction 95) -> (junction 98)
  data: PosAvlOut function_output; bk function_output; zero function_output; lgrstup function_output; lgrstin function_output; fwd function_output; IfVeSMSuSecRwLtStBkReclnUpwdDnwdPos input; IfVeSMSuSecRwLtStLgrstOtwdInwdPos input; IfVeSMSuSecRwLtStLgrstUpwdDnwdPos input; SecRwLtStBkReclnStgDone input; SecRwLtStFrwdBkwdStgDone input; SecRwLtStLgrstOtwdInwdStgDone input; SecRwLtStLgrstUpwdDnwdStgDone input; ThdRwLtStBkReclnStgDone input; ThdRwLtStFwdBkwdStgDone input; VIPLR2LBkReclnUpwdDnwdTrgtPos input; VIPLR2LLgrstInwdOtwdTrgtPos input; VIPLR2LLgrstUpwdDnwdTrgtPos input; SecRwLtStBkReclnEn output boolean; SecRwLtStFrwdBkwdEn output boolean; SecRwLtStLgrstOtwdInwdEn output boolean; ThdRwLtStBkReclnEn output boolean; ThdRwLtStFwdBkwdEn output boolean; SecRwLtStLgrstUpwdDnwdEn output boolean; ZeroLStgDone input; ZeroLEn output boolean; IfVeSMSuSecRwLtStZeroPos input; VIPLMdR2LZeroTrgtPos input; PosAvl output boolean; bktrgt local uint16; zerotrgt local uint16; lgrstuptrgt local uint16; lgrstintrgt local uint16; fwdtrgt local uint16; FirstTrig input boolean
  events: LgrstOpn output FUNCTION_CALL_EVENT
